simulink model "DashboardExample"  (R2025a)
settings: Solver=FixedStepAuto  StartTime=0.0  StopTime=inf  FixedStep=0.02  RelTol=1e-3  EnableMultiTasking=on
libraries: pingui x9, GenericTarget x2
settings Model: Creator=damerius  LastModifiedBy=damerius
settings SolverCC: ConcurrentTasks=on
settings DataIOCC: SaveOutput=off  SignalLogging=off  DSMLogging=off  SaveTime=off  ReturnWorkspaceOutputs=off
settings OptimizationCC: DefaultParameterBehavior=Inlined  ZeroExternalMemoryAtStartup=off  ZeroInternalMemoryAtStartup=off  SimCompilerOptimization=on
settings DebuggingCC: UnconnectedInputMsg=warning  UnconnectedOutputMsg=warning  UnconnectedLineMsg=warning
settings HardwareCC: ProdBitPerLong=64.0  ProdHWDeviceType=Intel->x86-64 (Linux 64)  TargetBitPerLong=64.0  TargetBitPerPointer=64.0  TargetBitPerSizeT=64.0  TargetBitPerPtrDiffT=64.0  TargetLargestAtomicFloat=Float  TargetIntDivRoundTo=Zero  TargetEndianess=LittleEndian  TargetWordSize=64.0  TargetHWDeviceType=Intel->x86-64 (Linux 64)  ProdEqTarget=off
settings ModelReferenceCC: EnableRefExpFcnMdlSchedulingChecks=on
settings SFSimCC: SimParseCustomCode=off  SimGenImportedTypeDefs=on  SimTargetLang=C++  SimDLTargetLibrary=mkl-dnn
settings RTWCC: GenCodeOnly=on  PackageGeneratedCodeAndArtifacts=on  PackageName=PackNGo  BuildConfiguration=Faster Runs  TargetLang=C++
settings CodeAppCC: ForceParamTrailComments=on  MaxIdLength=128.0  StateflowObjectComments=on  MATLABSourceComments=on  UseSimReservedNames=on
settings GRTTargetCC: TargetLangStandard=C++11 (ISO)  MatFileLogging=off  CodeInterfacePackaging=C++ class  SubcomponentCodeInterfacePackaging=C++ class

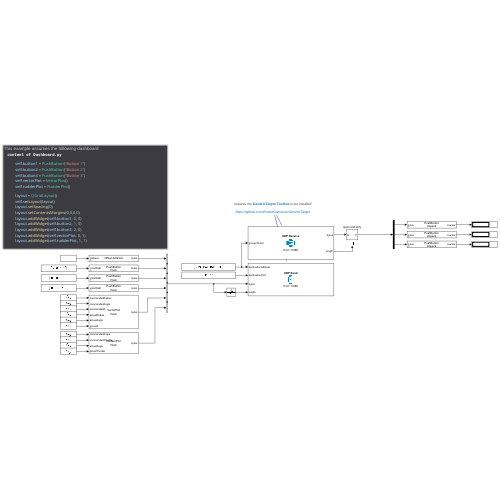
[thumbnail: Simulink's stored preview of the top-level diagram]
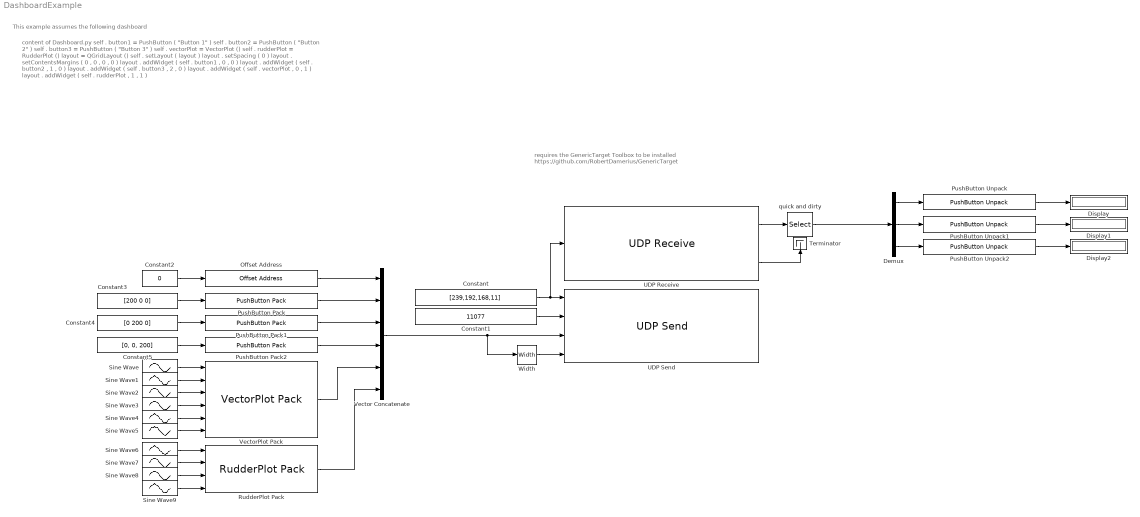
== system DashboardExample ==
  note: This example assumes the following dashboard
  note: content of Dashboard.py
      |
      | self . button1 = PushButton ( "Button 1" )
      | self . button2 = PushButton ( "Button 2" )
      | self . button3 = PushButton ( "Button 3" )
      | self . vectorPlot = VectorPlot ()
      | self . rudderPlot = RudderPlot ()
      |
      | layout = QGridLayout ()
      | self . setLayout ( layout )
      | layout . setSpacing ( 0 )
      | layout . setContentsMargins ( 0 , 0 , 0 , 0 )
      | layout . addWidget ( self . button1 , 0 , 0 )
      | layout . addWidget ( self . button2 , 1 , 0 )
      | layout . addWidget ( self . button3 , 2 , 0 )
      | layout . addWidget ( self . vectorPlot , 0 , 1 )
      | layout . addWidget ( self . rudderPlot , 1 , 1 )
  note: requires the GenericTarget Toolbox to be installed
      |
      | https://github.com/RobertDamerius/GenericTarget
  Constant : Constant  Value=[239,192,168,11]  OutDataTypeStr=uint8
  Constant1 : Constant  Value=11077  OutDataTypeStr=uint16
  Constant2 : Constant  Value=0  OutDataTypeStr=uint32
  Constant3 : Constant  Value=[200 0 0]  OutDataTypeStr=uint8
  Constant4 : Constant  Value=[0 200 0]  OutDataTypeStr=uint8
  Constant5 : Constant  Value=[0, 0, 200]  OutDataTypeStr=uint8
  Demux : Demux  Outputs=3
  Display : Display
  Display1 : Display
  Display2 : Display
  Offset Address : pingui/Offset Address
  PushButton Pack : pingui/PushButton Pack
  PushButton Pack1 : pingui/PushButton Pack
  PushButton Pack2 : pingui/PushButton Pack
  PushButton Unpack : pingui/PushButton Unpack
  PushButton Unpack1 : pingui/PushButton Unpack
  PushButton Unpack2 : pingui/PushButton Unpack
  RudderPlot Pack : pingui/RudderPlot Pack
  Sine Wave : Sin  SampleTime=0
  Sine Wave1 : Sin  Phase=2  SampleTime=0
  Sine Wave2 : Sin  Phase=1  SampleTime=0
  Sine Wave3 : Sin  Phase=0.1  SampleTime=0
  Sine Wave4 : Sin  Phase=2.1  SampleTime=0
  Sine Wave5 : Sin  Phase=1.1  SampleTime=0
  Sine Wave6 : Sin  Phase=2  SampleTime=0
  Sine Wave7 : Sin  SampleTime=0
  Sine Wave8 : Sin  Phase=2.1  SampleTime=0
  Sine Wave9 : Sin  Phase=0.1  SampleTime=0
  Terminator : Terminator
  UDP Receive : GenericTarget/Interface/UDP Receive  showDetails=off  localPort=11088  deviceName=''  rxBufferSize=2048  multicastGroupSource=external  multicastGroup=[0,0,0,0]  multicastTTL=1  multicastInterfaceAddress=[0,0,0,0]  multicastAll=on  multicastLoop=on  socketPriority=6  allowBroadcast=off  allowZeroLengthMessage=off  fetchAll=on  SampleTime=-1
      settings: SourceProductName=Generic Target
  UDP Send : GenericTarget/Interface/UDP Send  showDetails=off  localPort=11088  deviceName=''  multicastTTL=1  multicastInterfaceAddress=[0,0,0,0]  multicastAll=on  multicastLoop=on  socketPriority=6  allowBroadcast=off  allowZeroLengthMessage=off  SampleTime=-1
      settings: SourceProductName=Generic Target
  Vector Concatenate : Concatenate  NumInputs=6
  VectorPlot Pack : pingui/VectorPlot Pack
  Width : Width  DataType=uint32
  quick and dirty : Selector  IndexOptions=Index vector (dialog)  Indices=1:3  OutputSizes=1
  wires:
  Constant/1 -> UDP Receive/1, UDP Send/1
  Constant1/1 -> UDP Send/2
  UDP Receive/1 -> quick and dirty/1
  UDP Receive/2 -> Terminator/1
  quick and dirty/1 -> Demux/1
  Demux/1 -> PushButton Unpack/1
  Demux/2 -> PushButton Unpack1/1
  Demux/3 -> PushButton Unpack2/1
  PushButton Unpack/1 -> Display/1
  PushButton Unpack1/1 -> Display1/1
  PushButton Unpack2/1 -> Display2/1
  Constant2/1 -> Offset Address/1
  Offset Address/1 -> Vector Concatenate/1
  PushButton Pack/1 -> Vector Concatenate/2
  PushButton Pack1/1 -> Vector Concatenate/3
  PushButton Pack2/1 -> Vector Concatenate/4
  VectorPlot Pack/1 -> Vector Concatenate/5
  RudderPlot Pack/1 -> Vector Concatenate/6
  Vector Concatenate/1 -> Width/1, UDP Send/3
  Width/1 -> UDP Send/4
  Constant4/1 -> PushButton Pack1/1
  Constant5/1 -> PushButton Pack2/1
  Constant3/1 -> PushButton Pack/1
  Sine Wave/1 -> VectorPlot Pack/1
  Sine Wave1/1 -> VectorPlot Pack/2
  Sine Wave2/1 -> VectorPlot Pack/3
  Sine Wave3/1 -> VectorPlot Pack/4
  Sine Wave4/1 -> VectorPlot Pack/5
  Sine Wave5/1 -> VectorPlot Pack/6
  Sine Wave6/1 -> RudderPlot Pack/1
  Sine Wave7/1 -> RudderPlot Pack/2
  Sine Wave8/1 -> RudderPlot Pack/3
  Sine Wave9/1 -> RudderPlot Pack/4
